simulink model "BuckyWagon_01"  (Simulink 7.5)
settings: Solver=FixedStepDiscrete  StartTime=0.0  StopTime=10.0  RelTol=1e-3
PreLoadFcn:
  | try, eval([bdroot '_setup']); catch, eval('model_setup', ''); end
InitFcn:
  | try, eval([bdroot '_setup']); catch, eval('model_setup', ''); end
undefined symbols (not defined in the file or in its folder): ECU565, High, Low, miniviewSetup, motohawk_build_version, motohawk_get_faults, motohawk_setup_toolchains, motohawk_trunc_name, motohawk_vardec_config_group, motohawk_vardec_path, tc, True
libraries: MotoHawk_lib x406, simulink x30, miniview_lib x10, motohawk_control_primitives_lib x9, MotoHawk_VDOGauge_lib x8, motohawk_engine_lib x7, motohawk_annotations_lib x2
(part 3 of 7)

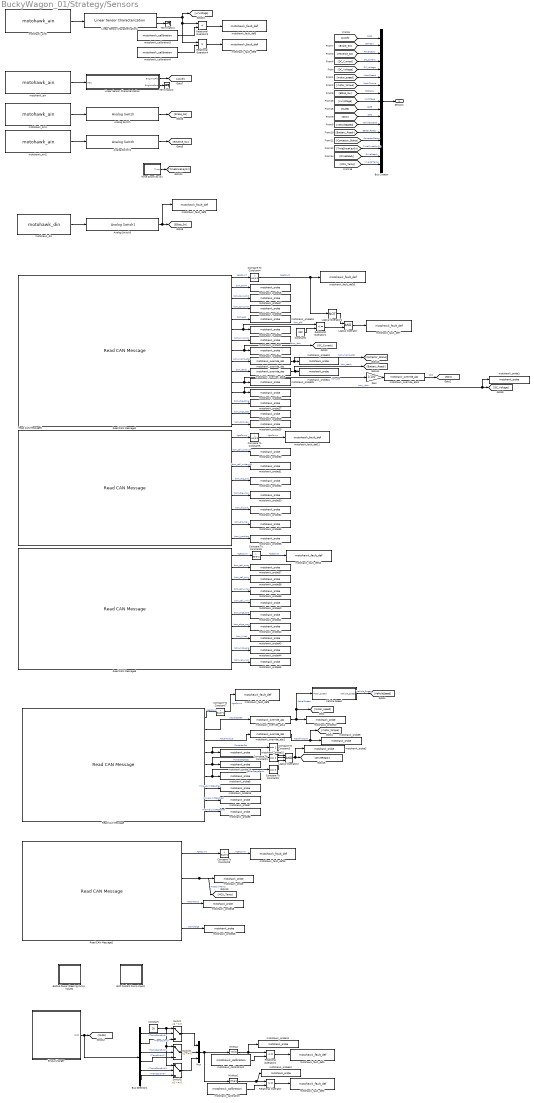
== system BuckyWagon_01/Strategy/Sensors ==
  Analog Switch : motohawk_engine_lib/Analog Switch  SystemSampleTime=-1  nam='Brake_Switch'  prefix='Brake_'  switchpoint=500  polarity=High-True  parent_group='Sensors | Brake'
  Analog Switch1 : motohawk_engine_lib/Analog Switch  SystemSampleTime=-1  nam='Reverse_Switch'  prefix='Reverse_'  switchpoint=500  polarity=Low-True  parent_group='Sensors | Reverse'
  Analog Switch3 : motohawk_engine_lib/Analog Switch1  SystemSampleTime=-1  nam='EStop_Switch'  prefix='EStop_'  polarity=Low-True  parent_group='Sensors | EStop'
  Brusa Charger : Subsystem  AncestorBlock=motohawk_annotations_lib/Display Image File  mask(Display Image File){image_file='NLG5.jpg'}
      mask prompts: image_file "Image File"
      mask help:
      | Enter an image file on the current MATLAB path to display on this block.
      |
      | Double-clicking this block opens the contents of the subsystem.  Right-click and select 'Mask parameters...' to select a new image file.
      |
      | To use just the mask of this block in a model, but supply your own contents, break the link to the library.
      mask init:
      | try,
      | 	img = imread(image_file);
      | 	motohawk_block_image(gcb, image_file);
      | catch,
      | 	img = imread('image_not_found.jpg');
      | end
      settings: OpenFcn=open_system(gcb,'force');  MoveFcn=motohawk_block_image(gcb, motohawk_get_param_ws(gcb, 'image_file'));
      mask Display: image(img);
  Bus Creator : BusCreator  Inputs=17
  Bus Selector1 : BusSelector  OutputSignals=Errors/Warnings.TempSensExt1,Temp.TempExtrn1,Errors/Warnings.TempSensExt2,Temp.TempExtrn2,Errors/Warnings.TempSensExt3,Temp.TempExtrn3
  Compare To Constant1 : simulink/Logic and Bit Operations/Compare To Constant  SystemSampleTime=-1  relop===  const=1  LogicOutDataTypeMode=boolean
  Compare To Constant3 : simulink/Logic and Bit Operations/Compare To Constant  SystemSampleTime=-1  relop===  const=1  LogicOutDataTypeMode=boolean
  Compare To Constant{4..8} (5 alike) : simulink/Logic and Bit Operations/Compare To Constant  SystemSampleTime=-1  relop=>  const=50/5*2  LogicOutDataTypeMode=boolean  ZeroCross=off
  Compare To Constant9 : simulink/Logic and Bit Operations/Compare To Constant  SystemSampleTime=-1  relop===  const=0  LogicOutDataTypeMode=boolean
  Constant : Constant  Value=20  OutDataType=sfix(16)  OutScaling=2^0
  Constant1 : Constant  Value=200  OutDataType=fixdt(1, 16)  OutScaling=2^0
  EHPAS Power Steering Pump Inputts : Subsystem  TreatAsAtomicUnit=on
  EMP Coolant Pump Inputs : Subsystem  TreatAsAtomicUnit=on
  Gain : Gain  Gain=1/100  ParameterDataType=fixdt(1, 16)  ParameterScaling=2^0  OutDataType=fixdt(1, 16)  OutScaling=2^0
  Linear Sensor Characterization : Subsystem  AncestorBlock=motohawk_engine_lib/Linear Sensor Characterization  mask(Linear Sensor Characterization){nam='Accel_Pedal', prefix='Accel_', units='%', inputunits='ADC', parent_group='Sensors | Accel', samp_time=0.005}
      mask prompts: nam "Name"; units "Output Units"; inputunits "Input Units"; parent_group "MotoTune Group"; samp_time "Sample Time"
      mask help:
      | Converts from A/D Counts to Engineering Units, using a Gain and Offset.
      | Saturates the converted value around Min and Max values, and triggers a Fault when out of range.
      mask init:
      | lbl = ['Linear Sensor: ' nam ' [' units ']'];
      | group = [parent_group ' | ' nam];
      settings: RTWSystemCode=Function  RTWFcnNameOpts=Use subsystem name  RTWFileNameOpts=Use function name
      mask Display:
      | patch([0 0 1 1], [0 0.075 0.075 0], [230/255 0/255 0/255])
      | patch([0 0 1 1], [0.025 0.05 0.05 0.025], [150/255 0/255 0/255])
      | patch([0 0 1 1], [0 0.025 0.025 0], [0/255 0/255 0/255])
      | 
      | disp(lbl);
  Linear Sensor Characterization1 : motohawk_engine_lib/Linear Sensor Characterization  SystemSampleTime=-1  nam='LVVolt'  prefix='LVVolt_'  units='V'  inputunits='ADC'  parent_group='Sensors | LVVolt'  samp_time=0.005
      link override First Order Low Pass/motohawk_calibration: val=0.01
      link override motohawk_calibration3: val=0.69
      link override motohawk_calibration4: val=0.041379
      link override motohawk_fault_def2: id=0
      link override motohawk_fault_def3: id=0
  Logical Operator : Logic  AllPortsSameDT=off  OutDataTypeMode=boolean  LogicDataType=fixdt(0, 8)  OutDataTypeStr=boolean
  Logical Operator1 : Logic  Operator=NOT  Inputs=1  AllPortsSameDT=off  OutDataTypeMode=boolean  LogicDataType=fixdt(0, 8)  OutDataTypeStr=boolean
  Logical Operator2 : Logic  Inputs=3  IconShape=distinctive  AllPortsSameDT=off  OutDataTypeMode=boolean  LogicDataType=fixdt(0, 8)  OutDataTypeStr=boolean
  MinMax : MinMax  OutDataType=sfix(16)  OutScaling=2^0
  MinMax1 : MinMax  Function=max  OutDataType=sfix(16)  OutScaling=2^0
  Mux : Mux  Inputs=3
  Read CAN Message : MotoHawk_lib/CAN Blocks/Read CAN Message  nam=['CAN_' num2str(2)]  bus=-2  msg=solectria_CANStatusID1  queue=1  slot=''  valid=off  stale=on  labelwires=on
  Read CAN Message1 : MotoHawk_lib/CAN Blocks/Read CAN Message  nam='CAN_2'  bus=-2  msg=BMS_A123_410  queue=1  slot=''  valid=off  stale=on  labelwires=on
  Read CAN Message2 : MotoHawk_lib/CAN Blocks/Read CAN Message  nam=['CAN_' num2str(2)]  bus=-2  msg=solectria_CANStatusID2  queue=1  slot=''  valid=off  stale=on  labelwires=on
  Read CAN Message5 : MotoHawk_lib/CAN Blocks/Read CAN Message  nam='CAN_2'  bus=-2  msg=BMS_A123_420  queue=1  slot=''  valid=off  stale=on  labelwires=on
  Read CAN Message6 : MotoHawk_lib/CAN Blocks/Read CAN Message  nam='CAN_2'  bus=-2  msg=BMS_A123_430  queue=1  slot=''  valid=off  stale=on  labelwires=on
  Relational Operator : RelationalOperator  LogicOutDataTypeMode=boolean  OutDataTypeStr=boolean
  Relational Operator1 : RelationalOperator  Operator=<=  LogicOutDataTypeMode=boolean  LogicDataType=fixdt(0, 8)  OutDataTypeStr=boolean
  Relational Operator2 : RelationalOperator  Operator=<=  LogicOutDataTypeMode=boolean  OutDataTypeStr=boolean
  Relational Operator3 : RelationalOperator  Operator=<  LogicOutDataTypeMode=boolean  OutDataTypeStr=boolean
  Relational Operator4 : RelationalOperator  Operator=>  LogicOutDataTypeMode=boolean  OutDataTypeStr=boolean
  Switch : Switch  Criteria=u2 ~= 0  OutDataType=sfix(16)  OutScaling=2^0
  Switch1 : Switch  Criteria=u2 ~= 0  OutDataType=sfix(16)  OutScaling=2^0
  Switch2 : Switch  Criteria=u2 ~= 0  OutDataType=sfix(16)  OutScaling=2^0
  Terminator2 : Terminator
  Terminator4 : Terminator
  Time Since Key On : Subsystem
  Vehicle Speed : Subsystem
  motohawk_ain : MotoHawk_lib/Analog I//O Blocks/motohawk_ain  res_name=[]  text_resource=AN4M  code_resource=NONE  val_resource=-1  target=ECU565-128  resource_enum_str=(None)=-1,ECUP=53,DRVP=54,XDRP=55,AN1M=56,AN2M=57,AN3M=58,AN4M=59,AN5M=60,AN6M=61,AN7M=62,AN8M=63,AN9M=64,AN10M=65,AN11M=66,AN12M=67,AN13M=68,AN14M=69,AN15M=70,AN16M=71,AN17M=72,AN18M=73,AN19M=74,AN20M=75,AN21M=76,AN22M=77,AN23M=78,AN24M=79,AN25M=80,AN26M=81,AN27M=82,AN28M=83,AN29M=84,AN30M=85,AN31M=86,AN32M=87,AN33M=88,AN34M=89,O2A=90,O2B=91,XDRP_B=92,REF_14V=143  altref=5V Reference  typ=uint16  num_adc_bits=10  use_stat=off  use_vardec=on  nam='Accel_Pedal_Pin'  read_level=1  write_level=1  group='System | I/O Pins | Inputs Config'
  motohawk_ain1 : MotoHawk_lib/Analog I//O Blocks/motohawk_ain  res_name=[]  text_resource=AN2M  code_resource=NONE  val_resource=-1  target=ECU565-128  resource_enum_str=(None)=-1,ECUP=53,DRVP=54,XDRP=55,AN1M=56,AN2M=57,AN3M=58,AN4M=59,AN5M=60,AN6M=61,AN7M=62,AN8M=63,AN9M=64,AN10M=65,AN11M=66,AN12M=67,AN13M=68,AN14M=69,AN15M=70,AN16M=71,AN17M=72,AN18M=73,AN19M=74,AN20M=75,AN21M=76,AN22M=77,AN23M=78,AN24M=79,AN25M=80,AN26M=81,AN27M=82,AN28M=83,AN29M=84,AN30M=85,AN31M=86,AN32M=87,AN33M=88,AN34M=89,O2A=90,O2B=91,XDRP_B=92,REF_14V=143  altref=5V Reference  typ=uint16  num_adc_bits=10  use_stat=off  use_vardec=on  nam='Brake_Switch_Pin'  read_level=1  write_level=1  group='System | I/O Pins | Inputs Config'
  motohawk_ain2 : MotoHawk_lib/Analog I//O Blocks/motohawk_ain  res_name=[]  text_resource=AN1M  code_resource=NONE  val_resource=-1  target=ECU565-128  resource_enum_str=(None)=-1,ECUP=53,DRVP=54,XDRP=55,AN1M=56,AN2M=57,AN3M=58,AN4M=59,AN5M=60,AN6M=61,AN7M=62,AN8M=63,AN9M=64,AN10M=65,AN11M=66,AN12M=67,AN13M=68,AN14M=69,AN15M=70,AN16M=71,AN17M=72,AN18M=73,AN19M=74,AN20M=75,AN21M=76,AN22M=77,AN23M=78,AN24M=79,AN25M=80,AN26M=81,AN27M=82,AN28M=83,AN29M=84,AN30M=85,AN31M=86,AN32M=87,AN33M=88,AN34M=89,O2A=90,O2B=91,XDRP_B=92,REF_14V=143  altref=5V Reference  typ=uint16  num_adc_bits=10  use_stat=off  use_vardec=on  nam='Reverse_Switch_Pin'  read_level=1  write_level=1  group='System | I/O Pins | Inputs Config'
  motohawk_ain5 : MotoHawk_lib/Analog I//O Blocks/motohawk_ain  res_name=[]  text_resource=DRVP  code_resource=NONE  val_resource=-1  target=ECU565-128  resource_enum_str=(None)=-1,ECUP=53,DRVP=54,XDRP=55,AN1M=56,AN2M=57,AN3M=58,AN4M=59,AN5M=60,AN6M=61,AN7M=62,AN8M=63,AN9M=64,AN10M=65,AN11M=66,AN12M=67,AN13M=68,AN14M=69,AN15M=70,AN16M=71,AN17M=72,AN18M=73,AN19M=74,AN20M=75,AN21M=76,AN22M=77,AN23M=78,AN24M=79,AN25M=80,AN26M=81,AN27M=82,AN28M=83,AN29M=84,AN30M=85,AN31M=86,AN32M=87,AN33M=88,AN34M=89,O2A=90,O2B=91,XDRP_B=92,REF_14V=143  altref=5V Reference  typ=uint16  num_adc_bits=10  use_stat=off  use_vardec=on  nam='LV_Voltage_Pin'  read_level=1  write_level=1  group='System | I/O Pins | Inputs Config'
  motohawk_calibration : MotoHawk_lib/Calibration & Probing Blocks/motohawk_calibration  nam='BattOverTemp_Pt'  val=70  storage=Calibration  show_more=on  name_source=Use Parameter  data_type=Inherit from 'Default Value'  read_level=1  write_level=1  ovr_cals=on  view_as=Number  enum_struct={'Disabled', 'Enabled'}  vector_style=Wide Row  use_help_units=on  help='Temperature at which an overtemp fault occurs'  units='C'  use_header_enum=off  row_header_enum={}  col_header_enum={}  use_min_max=off  min_val=-inf  max_val=inf  use_precision=off  precision=''  gain=1  offset=0  exp=1  use_mototune_group=on  mototune_group='Sensors | Brusa'
  motohawk_calibration2 : MotoHawk_lib/Calibration & Probing Blocks/motohawk_calibration  nam='BattUnderTemp_Pt'  val=-40  storage=Calibration  show_more=on  name_source=Use Parameter  data_type=Inherit from 'Default Value'  read_level=1  write_level=1  ovr_cals=on  view_as=Number  enum_struct={'Disabled', 'Enabled'}  vector_style=Wide Row  use_help_units=on  help='Temperature at which an overtemp fault occurs'  units='C'  use_header_enum=off  row_header_enum={}  col_header_enum={}  use_min_max=off  min_val=-inf  max_val=inf  use_precision=off  precision=''  gain=1  offset=0  exp=1  use_mototune_group=on  mototune_group='Sensors | Brusa'
  motohawk_calibration3 : MotoHawk_lib/Calibration & Probing Blocks/motohawk_calibration  nam='Low12VThres'  val=12.8  storage=Calibration  show_more=on  name_source=Use Parameter  data_type=Inherit from 'Default Value'  read_level=1  write_level=1  ovr_cals=on  view_as=Number  enum_struct={'Disabled', 'Enabled'}  vector_style=Wide Row  use_help_units=on  help='Voltage below with low 12V fault occurs.'  units='V'  use_header_enum=off  row_header_enum={}  col_header_enum={}  use_min_max=off  min_val=-inf  max_val=inf  use_precision=on  precision=''  gain=1  offset=0  exp=1  use_mototune_group=on  mototune_group='Sensors | LVVolt'
  motohawk_calibration4 : MotoHawk_lib/Calibration & Probing Blocks/motohawk_calibration  nam='High12VThres'  val=14.5  storage=Calibration  show_more=on  name_source=Use Parameter  data_type=Inherit from 'Default Value'  read_level=1  write_level=1  ovr_cals=on  view_as=Number  enum_struct={'Disabled', 'Enabled'}  vector_style=Wide Row  use_help_units=on  help='Voltage below with low 12V fault occurs.'  units='V'  use_header_enum=off  row_header_enum={}  col_header_enum={}  use_min_max=off  min_val=-inf  max_val=inf  use_precision=on  precision=''  gain=1  offset=0  exp=1  use_mototune_group=on  mototune_group='Sensors | LVVolt'
  motohawk_din : MotoHawk_lib/Digital I//O Blocks/motohawk_din  resource_name=[]  text_resource=(None)  code_resource=RES_AN1M  val_resource=-1  target=ECU565-128  resource_enum_str=(None)=-1,AN1M=56,AN2M=57,AN3M=58,AN4M=59,AN5M=60,AN6M=61,AN7M=62,AN8M=63,AN9M=64,AN10M=65,AN11M=66,AN12M=67,AN13M=68,AN14M=69,AN15M=70,AN16M=71,AN17M=72,AN18M=73,AN19M=74,AN20M=75,AN21M=76,AN22M=77,AN23M=78,AN24M=79,AN25M=80,AN26M=81,AN27M=82,AN28M=83,AN29M=84,AN30M=85,AN31M=86,AN32M=87,AN33M=88,AN34M=89,O2A=90,O2B=91,DG1M=93,DG2M=94,DG3M=95,DG4M=96,DG5M=102,DG6M=103,DG7M=104,SPD1=105,SPD2=106,DG8M=111  pullup=None  use_stat=off  use_vardec=on  nam='EStop_Switch_Pin'  read_level=1  write_level=1  group='System | I/O Pins | Inputs Config'
  motohawk_fault_def10 : MotoHawk_lib/Fault Management Blocks/motohawk_fault_def  nam='NoCAN_BCM_410'  mode=Enabled  id=0  x=10  y=20  input_suspected=on  indeterminate=off  increment_xy=on  downsample_count=1  ovr_cals=on  ovr_actions=on  show_actions=off  action1_name=''  action1_cond=(None)  action2_name=''  action2_cond=(None)  action3_name=''  action3_cond=(None)  action4_name=''  action4_cond=(None)
  motohawk_fault_def11 : MotoHawk_lib/Fault Management Blocks/motohawk_fault_def  nam='NoCAN_BCM_420'  mode=Enabled  id=0  x=10  y=20  input_suspected=on  indeterminate=off  increment_xy=on  downsample_count=1  ovr_cals=on  ovr_actions=on  show_actions=off  action1_name=''  action1_cond=(None)  action2_name=''  action2_cond=(None)  action3_name=''  action3_cond=(None)  action4_name=''  action4_cond=(None)
  motohawk_fault_def12 : MotoHawk_lib/Fault Management Blocks/motohawk_fault_def  nam='NoCAN_BCM_430'  mode=Enabled  id=0  x=10  y=20  input_suspected=on  indeterminate=off  increment_xy=on  downsample_count=1  ovr_cals=on  ovr_actions=on  show_actions=off  action1_name=''  action1_cond=(None)  action2_name=''  action2_cond=(None)  action3_name=''  action3_cond=(None)  action4_name=''  action4_cond=(None)
  motohawk_fault_def13 : MotoHawk_lib/Fault Management Blocks/motohawk_fault_def  nam='NoCAN_Solectria_462'  mode=Enabled  id=[]  x=50/5  y=50/5*2  input_suspected=on  indeterminate=off  increment_xy=on  downsample_count=1  ovr_cals=on  ovr_actions=on  show_actions=off  action1_name=''  action1_cond=(None)  action2_name=''  action2_cond=(None)  action3_name=''  action3_cond=(None)  action4_name=''  action4_cond=(None)
  motohawk_fault_def2 : MotoHawk_lib/Fault Management Blocks/motohawk_fault_def  nam='BattOverTemp'  mode=Disabled  id=0  x=25  y=50  input_suspected=on  indeterminate=off  increment_xy=on  downsample_count=1  ovr_cals=on  ovr_actions=on  show_actions=off  action1_name=''  action1_cond=(None)  action2_name=''  action2_cond=(None)  action3_name=''  action3_cond=(None)  action4_name=''  action4_cond=(None)
  motohawk_fault_def3 : MotoHawk_lib/Fault Management Blocks/motohawk_fault_def  nam='ESTOPped'  mode=Sticky  id=0  x=50  y=100  input_suspected=on  indeterminate=off  increment_xy=on  downsample_count=1  ovr_cals=on  ovr_actions=on  show_actions=off  action1_name='DisableDrive'  action1_cond=Active  action2_name=''  action2_cond=(None)  action3_name=''  action3_cond=(None)  action4_name=''  action4_cond=(None)
  motohawk_fault_def4 : MotoHawk_lib/Fault Management Blocks/motohawk_fault_def  nam='BattUnderTemp'  mode=Disabled  id=0  x=25  y=50  input_suspected=on  indeterminate=off  increment_xy=on  downsample_count=1  ovr_cals=on  ovr_actions=on  show_actions=off  action1_name=''  action1_cond=(None)  action2_name=''  action2_cond=(None)  action3_name=''  action3_cond=(None)  action4_name=''  action4_cond=(None)
  motohawk_fault_def5 : MotoHawk_lib/Fault Management Blocks/motohawk_fault_def  nam='LVVoltLow'  mode=Enabled  id=0  x=100  y=200  input_suspected=on  indeterminate=off  increment_xy=on  downsample_count=1  ovr_cals=on  ovr_actions=on  show_actions=off  action1_name=''  action1_cond=(None)  action2_name=''  action2_cond=(None)  action3_name=''  action3_cond=(None)  action4_name=''  action4_cond=(None)
  motohawk_fault_def6 : MotoHawk_lib/Fault Management Blocks/motohawk_fault_def  nam='LVVoltHigh'  mode=Enabled  id=0  x=25  y=50  input_suspected=on  indeterminate=off  increment_xy=on  downsample_count=1  ovr_cals=on  ovr_actions=on  show_actions=off  action1_name=''  action1_cond=(None)  action2_name=''  action2_cond=(None)  action3_name=''  action3_cond=(None)  action4_name=''  action4_cond=(None)
  motohawk_fault_def7 : MotoHawk_lib/Fault Management Blocks/motohawk_fault_def  nam='GroundFlt'  mode=Sticky  id=0  x=25  y=50  input_suspected=on  indeterminate=off  increment_xy=on  downsample_count=1  ovr_cals=on  ovr_actions=on  show_actions=off  action1_name='EmergencyShutdown'  action1_cond=Active  action2_name=''  action2_cond=(None)  action3_name=''  action3_cond=(None)  action4_name=''  action4_cond=(None)
  motohawk_fault_def8 : MotoHawk_lib/Fault Management Blocks/motohawk_fault_def  nam='NoCAN_Solectria_461'  mode=Enabled  id=[]  x=50/5  y=50/5*2  input_suspected=on  indeterminate=off  increment_xy=on  downsample_count=1  ovr_cals=on  ovr_actions=on  show_actions=off  action1_name=''  action1_cond=(None)  action2_name=''  action2_cond=(None)  action3_name=''  action3_cond=(None)  action4_name=''  action4_cond=(None)
  motohawk_override_abs : MotoHawk_lib/Calibration & Probing Blocks/motohawk_override_abs  SystemSampleTime=-1  parent_name='bcm_mainc_stat'  parent_val=0  show_more=on  name_source=Use Parameter  parent_read_level=1  parent_override_level=1  view_as=Number  enum_struct={'Disabled', 'Enabled'}  use_help_units=off  parent_help=''  parent_units=''  use_min_max=off  parent_min=-inf  parent_max=inf  use_precision=off  parent_precision=''  parent_gain=1  parent_offset=0  parent_exp=1  use_mototune_group=on  parent_group='Sensors | BCM'
  motohawk_override_abs1 : MotoHawk_lib/Calibration & Probing Blocks/motohawk_override_abs  SystemSampleTime=-1  parent_name='Override_Absolute'  parent_val=0  show_more=on  name_source=Use Input Wire Name  parent_read_level=1  parent_override_level=1  view_as=Number  enum_struct={'Disabled', 'Enabled'}  use_help_units=off  parent_help=''  parent_units=''  use_min_max=off  parent_min=-inf  parent_max=inf  use_precision=off  parent_precision=''  parent_gain=1  parent_offset=0  parent_exp=1  use_mototune_group=on  parent_group='Sensors | Solectria'
  motohawk_override_abs2 : MotoHawk_lib/Calibration & Probing Blocks/motohawk_override_abs  SystemSampleTime=-1  parent_name='Override_Absolute'  parent_val=0  show_more=on  name_source=Use Input Wire Name  parent_read_level=1  parent_override_level=1  view_as=Number  enum_struct={'Disabled', 'Enabled'}  use_help_units=off  parent_help=''  parent_units=''  use_min_max=off  parent_min=-inf  parent_max=inf  use_precision=off  parent_precision=''  parent_gain=1  parent_offset=0  parent_exp=1  use_mototune_group=on  parent_group='Sensors | Solectria'
  motohawk_override_abs4 : MotoHawk_lib/Calibration & Probing Blocks/motohawk_override_abs  SystemSampleTime=-1  parent_name='SOC'  parent_val=0.5  show_more=on  name_source=Use Parameter  parent_read_level=1  parent_override_level=1  view_as=Number  enum_struct={'Disabled', 'Enabled'}  use_help_units=off  parent_help=''  parent_units=''  use_min_max=on  parent_min=0  parent_max=1  use_precision=off  parent_precision=''  parent_gain=1  parent_offset=0  parent_exp=1  use_mototune_group=on  parent_group='Sensors | BCM'
  motohawk_override_abs5 : MotoHawk_lib/Calibration & Probing Blocks/motohawk_override_abs  SystemSampleTime=-1  parent_name='bcm_ready'  parent_val=0  show_more=on  name_source=Use Parameter  parent_read_level=1  parent_override_level=1  view_as=Number  enum_struct={'Disabled', 'Enabled'}  use_help_units=off  parent_help=''  parent_units=''  use_min_max=off  parent_min=-inf  parent_max=inf  use_precision=off  parent_precision=''  parent_gain=1  parent_offset=0  parent_exp=1  use_mototune_group=on  parent_group='Sensors | BCM'
  motohawk_probe{,6..8,13..15,48} (8 alike) : MotoHawk_lib/Calibration & Probing Blocks/motohawk_probe  nam='Probe'  show_more=on  name_source=Use Input Wire Name  read_level=1  view_as=Number  enum_struct={'Disabled', 'Enabled'}  vector_style=Wide Row  use_help_units=off  help=''  units=''  use_header_enum=off  row_header_enum={}  col_header_enum={}  use_precision=off  precision=''  gain=1  offset=0  exp=1  use_mototune_group=on  mototune_group='Sensors | Solectria'
  motohawk_probe1 : MotoHawk_lib/Calibration & Probing Blocks/motohawk_probe  nam='DC_Voltage'  show_more=on  name_source=Use Parameter  read_level=1  view_as=Number  enum_struct={'Disabled', 'Enabled'}  vector_style=Wide Row  use_help_units=off  help=''  units=''  use_header_enum=off  row_header_enum={}  col_header_enum={}  use_precision=off  precision=''  gain=1  offset=0  exp=1  use_mototune_group=on  mototune_group='Sensors'
  motohawk_probe10 : MotoHawk_lib/Calibration & Probing Blocks/motohawk_probe  nam='Probe'  show_more=on  name_source=Use Input Wire Name  read_level=1  view_as=Number  enum_struct={'Disabled', 'Enabled'}  vector_style=Wide Row  use_help_units=off  help=''  units=''  use_header_enum=off  row_header_enum={}  col_header_enum={}  use_precision=off  precision=''  gain=1  offset=0  exp=1  use_mototune_group=on  mototune_group='Sensors'
  motohawk_probe11 : MotoHawk_lib/Calibration & Probing Blocks/motohawk_probe  nam='BattMinTemp'  show_more=on  name_source=Use Parameter  read_level=1  view_as=Number  enum_struct={'Disabled', 'Enabled'}  vector_style=Wide Row  use_help_units=off  help=''  units=''  use_header_enum=off  row_header_enum={}  col_header_enum={}  use_precision=off  precision=''  gain=1  offset=0  exp=1  use_mototune_group=on  mototune_group='Sensors | Brusa'
  motohawk_probe12 : MotoHawk_lib/Calibration & Probing Blocks/motohawk_probe  nam='BattMaxTemp'  show_more=on  name_source=Use Parameter  read_level=1  view_as=Number  enum_struct={'Disabled', 'Enabled'}  vector_style=Wide Row  use_help_units=off  help=''  units=''  use_header_enum=off  row_header_enum={}  col_header_enum={}  use_precision=off  precision=''  gain=1  offset=0  exp=1  use_mototune_group=on  mototune_group='Sensors | Brusa'
  motohawk_probe{16..45} (30 alike) : MotoHawk_lib/Calibration & Probing Blocks/motohawk_probe  nam='Probe'  show_more=on  name_source=Use Input Wire Name  read_level=1  view_as=Number  enum_struct={'Disabled', 'Enabled'}  vector_style=Wide Row  use_help_units=off  help=''  units=''  use_header_enum=off  row_header_enum={}  col_header_enum={}  use_precision=off  precision=''  gain=1  offset=0  exp=1  use_mototune_group=on  mototune_group='Sensors | BCM'
  motohawk_probe2 : MotoHawk_lib/Calibration & Probing Blocks/motohawk_probe  nam='DriveReady'  show_more=on  name_source=Use Parameter  read_level=1  view_as=Number  enum_struct={'Disabled', 'Enabled'}  vector_style=Wide Row  use_help_units=off  help=''  units=''  use_header_enum=off  row_header_enum={}  col_header_enum={}  use_precision=off  precision=''  gain=1  offset=0  exp=1  use_mototune_group=on  mototune_group='Sensors'
  motohawk_probe46 : MotoHawk_lib/Calibration & Probing Blocks/motohawk_probe  nam='DCVoltage_Solectria'  show_more=on  name_source=Use Parameter  read_level=1  view_as=Number  enum_struct={'Disabled', 'Enabled'}  vector_style=Wide Row  use_help_units=off  help=''  units=''  use_header_enum=off  row_header_enum={}  col_header_enum={}  use_precision=off  precision=''  gain=1  offset=0  exp=1  use_mototune_group=on  mototune_group='Sensors | Solectria'
  motohawk_probe9 : MotoHawk_lib/Calibration & Probing Blocks/motohawk_probe  nam='Probe'  show_more=on  name_source=Use Input Wire Name  read_level=1  view_as=Number  enum_struct={'Disabled', 'Enabled'}  vector_style=Wide Row  use_help_units=off  help=''  units=''  use_header_enum=off  row_header_enum={}  col_header_enum={}  use_precision=off  precision=''  gain=1  offset=0  exp=1  use_mototune_group=on  mototune_group='Sensors'
  Sensors : Outport  OutDataType=sfix(16)  OutScaling=2^0
  wires:
  motohawk_ain/1 -> Linear Sensor Characterization/1(ADC)
  motohawk_ain1/1 -> Analog Switch/1
  Analog Switch/1 -> [Brake_Sw]
  Linear Sensor Characterization/1(EngUnitsFilt) -> [Accel]
  Linear Sensor Characterization/2(EngUnitsRaw) -> Terminator2/1
  Bus Creator/1 -> Sensors/1
  [Accel] -> Bus Creator/1  "Accel"
  [Brake_Sw] -> Bus Creator/2  "BrakeSw"
  [Reverse_Sw] -> Bus Creator/3  "ReverseSw"
  motohawk_ain2/1 -> Analog Switch1/1
  Analog Switch1/1 -> [Reverse_Sw]
  motohawk_din/1 -> Analog Switch3/1
  Analog Switch3/1 -> [EStop_Sw], motohawk_fault_def3/1
  motohawk_ain5/1 -> Linear Sensor Characterization1/1
  Linear Sensor Characterization1/2 -> Terminator4/1
  motohawk_calibration3/1 -> Relational Operator3/2
  Linear Sensor Characterization1/1 -> [LVVoltage], Relational Operator3/1, Relational Operator4/1
  Relational Operator3/1 -> motohawk_fault_def5/1
  motohawk_calibration4/1 -> Relational Operator4/2
  Relational Operator4/1 -> motohawk_fault_def6/1
  [DC_Current] -> Bus Creator/4  "DC_Current"
  [DC_Voltage] -> Bus Creator/5  "DC_Voltage"
  [motor_speed] -> Bus Creator/6  "MotorSpeed"
  [motor_torque] -> Bus Creator/7  "MotorTorque"
  [EStop_Sw] -> Bus Creator/8  "EStopSw"
  [LVVoltage] -> Bus Creator/9  "LVVoltage"
  [NLG5] -> Bus Creator/10  "NLG5"
  [SOC] -> Bus Creator/11  "SOC"
  [VehicleSpeed] -> Bus Creator/12  "VehicleSpeed"
  [Contactor_Status] -> Bus Creator/14  "ContactorStatus"
  [Battery_Ready] -> Bus Creator/13  "BatteryReady"
  Time Since Key On/1(Time) -> [TimeSinceKeyOn]
  [TimeSinceKeyOn] -> Bus Creator/15  "TimeSinceKeyOn"
  [DriveReady] -> Bus Creator/16  "DriveReady"
  [MCU_Temp] -> Bus Creator/17  "InverterTemp"
  Read CAN Message1/2 -> motohawk_probe16/1  "bcm_alarm"
  Read CAN Message1/3 -> motohawk_probe17/1  "bcm_cpwr_cmd"
  Read CAN Message1/4 -> motohawk_probe18/1  "bcm_cpwr_mon"
  Read CAN Message1/5 -> motohawk_probe19/1  "bcm_epo"
  Read CAN Message1/6 -> motohawk_probe20/1, Relational Operator1/1  "bcm_gfd"
  Read CAN Message1/7 -> motohawk_probe21/1  "bcm_hvil_mon"
  Read CAN Message1/8 -> motohawk_probe22/1, [DC_Current]  "bcm_ibat"
  Read CAN Message1/9 -> motohawk_override_abs/1  "bcm_mainc_stat"
  Read CAN Message1/10 -> motohawk_override_abs5/1  "bcm_ready"
  Read CAN Message1/11 -> motohawk_probe25/1, Gain/1  "bcm_soc"
  Read CAN Message1/12 -> motohawk_probe26/1, [DC_Voltage], motohawk_probe1/1  "bcm_vbat"
  Read CAN Message1/13 -> motohawk_probe27/1  "bcm_chg_done"
  Read CAN Message1/14 -> motohawk_probe28/1  "bcm_chgc_stat"
  Read CAN Message1/15 -> motohawk_probe29/1  "bcm_cool_req"
  Read CAN Message5/2 -> motohawk_probe30/1  "bcm_cell_overvolt"
  Read CAN Message5/3 -> motohawk_probe31/1  "bcm_cell_undervolt"
  Read CAN Message5/4 -> motohawk_probe32/1  "bcm_chg_buf"
  Read CAN Message5/5 -> motohawk_probe33/1  "bcm_chg_max"
  Read CAN Message5/6 -> motohawk_probe34/1  "bcm_dis_buf"
  Read CAN Message5/7 -> motohawk_probe35/1  "bcm_dis_max"
  Read CAN Message5/8 -> motohawk_probe36/1  "bcm_t_coolant"
  Read CAN Message6/2 -> motohawk_probe37/1  "bcm_cell_tmax"
  Read CAN Message6/3 -> motohawk_probe38/1  "bcm_cell_tmin"
  Read CAN Message6/4 -> motohawk_probe39/1  "bcm_cell_vmax"
  Read CAN Message6/5 -> motohawk_probe40/1  "bcm_cell_vmin"
  Read CAN Message6/6 -> motohawk_probe41/1  "bcm_chga_ena"
  Read CAN Message6/7 -> motohawk_probe42/1  "bcm_chga_mon"
  Read CAN Message6/8 -> motohawk_probe43/1  "bcm_lvbat"
  Read CAN Message6/9 -> motohawk_probe44/1  "bcm_mod_ena"
  Read CAN Message6/10 -> motohawk_probe45/1  "bcm_veh_mon"
  Compare To Constant4/1 -> motohawk_fault_def10/1, Logical Operator1/1  "AgeCount"
  Read CAN Message1/1 -> Compare To Constant4/1  "AgeCount"
  Compare To Constant5/1 -> motohawk_fault_def11/1  "AgeCount"
  Read CAN Message5/1 -> Compare To Constant5/1  "AgeCount"
  Compare To Constant6/1 -> motohawk_fault_def12/1  "AgeCount"
  Read CAN Message6/1 -> Compare To Constant6/1  "AgeCount"
  Constant1/1 -> Relational Operator1/2
  motohawk_override_abs4/1 -> [SOC]  "SOC"
  Gain/1 -> motohawk_override_abs4/1
  Relational Operator1/1 -> Logical Operator/2
  Logical Operator/1 -> motohawk_fault_def7/1
  Logical Operator1/1 -> Logical Operator/1
  motohawk_override_abs/1 -> motohawk_probe23/1, [Contactor_Status]  "bcm_mainc_stat"
  motohawk_override_abs5/1 -> [Battery_Ready], motohawk_probe24/1  "bcm_ready"
  Read CAN Message/3 -> motohawk_override_abs2/1  "ActualTorque"
  Read CAN Message/4 -> motohawk_probe15/1, Compare To Constant3/1  "ContactorSts"
  Read CAN Message/5 -> motohawk_probe14/1, Compare To Constant1/1  "PowerStageSts"
  Read CAN Message/6 -> motohawk_probe8/1, Compare To Constant9/1  "PowerStageFault"
  Read CAN Message/7 -> motohawk_probe13/1  "TorqueLimitReached"
  Read CAN Message/8 -> motohawk_probe7/1  "PowerLimitReached"
  Read CAN Message/9 -> motohawk_probe6/1  "ThermalLimitReached"
  Read CAN Message/1 -> Compare To Constant7/1  "AgeCount"
  Compare To Constant7/1 -> motohawk_fault_def8/1  "AgeCount"
  Read CAN Message2/2 -> motohawk_probe/1, [MCU_Temp]  "HeatsinkTemp"
  Read CAN Message2/3 -> motohawk_probe48/1  "MotorTemp"
  Read CAN Message2/1 -> Compare To Constant8/1  "AgeCount"
  motohawk_override_abs1/1 -> motohawk_probe10/1, [motor_speed], Vehicle Speed/1(Motor_Speed)  "ActualSpeed"
  Vehicle Speed/1(Vehicle_Speed) -> [VehicleSpeed]  "Vehicle_Speed"
  Read CAN Message/2 -> motohawk_override_abs1/1  "ActualSpeed"
  motohawk_override_abs2/1 -> motohawk_probe9/1, [motor_torque]  "ActualTorque"
  Read CAN Message2/4 -> motohawk_probe46/1  "DCVoltage"
  Compare To Constant8/1 -> motohawk_fault_def13/1  "AgeCount"
  Compare To Constant1/1 -> Logical Operator2/2
  Compare To Constant3/1 -> Logical Operator2/1
  Compare To Constant9/1 -> Logical Operator2/3
  Logical Operator2/1 -> [DriveReady], motohawk_probe2/1
  Brusa Charger/1(Out1) -> [NLG5], Bus Selector1/1
  MinMax1/1 -> Relational Operator/1, motohawk_probe12/1
  motohawk_calibration/1 -> Relational Operator/2
  Relational Operator/1 -> motohawk_fault_def2/1
  MinMax/1 -> Relational Operator2/1, motohawk_probe11/1
  motohawk_calibration2/1 -> Relational Operator2/2
  Relational Operator2/1 -> motohawk_fault_def4/1
  Bus Selector1/1 -> Switch/2  "<TempSensExt1>"
  Bus Selector1/2 -> Switch/3  "<TempExtrn1>"
  Bus Selector1/3 -> Switch1/2  "<TempSensExt2>"
  Bus Selector1/4 -> Switch1/3  "<TempExtrn2>"
  Bus Selector1/5 -> Switch2/2  "<TempSensExt3>"
  Bus Selector1/6 -> Switch2/3  "<TempExtrn3>"
  Constant/1 -> Switch/1, Switch1/1, Switch2/1
  Switch/1 -> Mux/1
  Switch1/1 -> Mux/2
  Switch2/1 -> Mux/3
  Mux/1 -> MinMax/1, MinMax1/1

== system BuckyWagon_01/Main Power Relay/Background/Delay ==
  note: Delay the rising and falling of a boolean signal
  In : Inport  OutDataType=sfix(16)  OutScaling=2^0
  Constant1 : Constant  Value=0  OutDataType=sfix(16)  OutScaling=2^0  OutDataTypeStr=Inherit: Inherit via back propagation
  Constant2 : Constant  Value=uint16( on_delay_count )  OutDataType=sfix(16)  OutScaling=2^0
  Constant3 : Constant  Value=0  OutDataType=sfix(16)  OutScaling=2^0  OutDataTypeStr=Inherit: Inherit via back propagation
  Constant4 : Constant  Value=uint16( off_delay_count )  OutDataType=sfix(16)  OutScaling=2^0
  Data Type Conversion : DataTypeConversion  RndMeth=Zero
  Data Type Conversion1 : DataTypeConversion  RndMeth=Zero
  Logical Operator : Logic  Operator=NOT  OutDataTypeMode=boolean  OutDataTypeStr=boolean
  Logical Operator1 : Logic  OutDataTypeMode=boolean  OutDataTypeStr=boolean
  Logical Operator2 : Logic  OutDataTypeMode=boolean  OutDataTypeStr=boolean
  MotoHawk S-R Flip-Flop : Subsystem  mask(MotoHawk S-R Flip-Flop){ic_bool=false}
      mask prompts: ic_bool "Initial condition Q (boolean)"
      mask help:
      | When input S (set) is TRUE, output Q is TRUE (and latched until reset).
      | When input R (reset) is TRUE, output Q is FALSE (and latched until set).
      | If both inputs S and R are TRUE, output Q is FALSE (reset wins).
      mask Display:
      | patch([0 0 1 1], [0 0.075 0.075 0], [230/255 0/255 0/255]);
      | patch([0 0 1 1], [0.025 0.05 0.05 0.025], [150/255 0/255 0/255]);
      | patch([0 0 1 1], [0 0.025 0.025 0], [0/255 0/255 0/255])
  Relational Operator1 : RelationalOperator  LogicOutDataTypeMode=boolean  OutDataTypeStr=boolean  ZeroCross=off  InputSameDT=on
  Relational Operator2 : RelationalOperator  LogicOutDataTypeMode=boolean  OutDataTypeStr=boolean  ZeroCross=off  InputSameDT=on
  Sum : Sum  Inputs=++|  OutDataType=sfix(16)  OutScaling=2^0  RndMeth=Zero  SaturateOnIntegerOverflow=on  InputSameDT=on
  Sum1 : Sum  Inputs=++|  OutDataType=sfix(16)  OutScaling=2^0  RndMeth=Zero  SaturateOnIntegerOverflow=on  InputSameDT=on
  Switch : Switch  Criteria=u2 ~= 0  Threshold=1  RndMeth=Zero  ZeroCross=off  InputSameDT=on
  Switch1 : Switch  Criteria=u2 ~= 0  Threshold=1  RndMeth=Zero  ZeroCross=off  InputSameDT=on
  Terminator : Terminator
  Unit Delay : UnitDelay  SampleTime=-1
  Unit Delay1 : UnitDelay  SampleTime=-1
  Out : Outport
  wires:
  Logical Operator1/1 -> MotoHawk S-R Flip-Flop/2(R)
  Logical Operator2/1 -> MotoHawk S-R Flip-Flop/1(S)
  Relational Operator1/1 -> Logical Operator2/2
  Relational Operator2/1 -> Logical Operator1/2
  MotoHawk S-R Flip-Flop/2(!Q) -> Terminator/1
  MotoHawk S-R Flip-Flop/1(Q) -> Out/1
  Constant4/1 -> Relational Operator2/2
  Logical Operator/1 -> Logical Operator1/1, Switch1/2, Data Type Conversion1/1
  Data Type Conversion1/1 -> Sum1/2  "0 to 1"
  Sum1/1 -> Switch1/1  "0 to 65535 (saturate hi)"
  Constant3/1 -> Switch1/3
  Switch1/1 -> Relational Operator2/1, Unit Delay1/1  "0 to 65535"
  In/1 -> Logical Operator/1, Logical Operator2/1, Switch/2, Data Type Conversion/1
  Data Type Conversion/1 -> Sum/2  "0 to 1"
  Sum/1 -> Switch/1  "0 to 65535 (saturate hi)"
  Constant1/1 -> Switch/3
  Switch/1 -> Unit Delay/1, Relational Operator1/1  "0 to 65535"
  Constant2/1 -> Relational Operator1/2
  Unit Delay1/1 -> Sum1/1  "0 to 65535"
  Unit Delay/1 -> Sum/1  "0 to 65535"

== system BuckyWagon_01/Main Power Relay/Background/Post Shutdown two ticks before MPRD off ==
  Trigger : TriggerPort  TriggerType=falling
  Function-Call Generator : simulink/Ports & Subsystems/Function-Call Generator  sample_time=-1  numberOfIterations=1
  Post Shutdown two ticks before MPRD off : MotoHawk_lib/Trigger Blocks/motohawk_event_call  SystemSampleTime=-1  mode=Post Event  trigger=SHUTDOWN_EVENT  target=ECU565_128
  motohawk_code_coverage : MotoHawk_lib/Extra Development Blocks/motohawk_code_coverage
  wires:
  Function-Call Generator/1 -> Post Shutdown two ticks before MPRD off/Trigger

== system BuckyWagon_01/Main Power Relay/Background/Processor Reboot ==
  Enable : EnablePort
  Trigger : TriggerPort  TriggerType=falling
  Force Module Reset : MotoHawk_lib/Extra Development Blocks/Force Module Reset
  motohawk_code_coverage : MotoHawk_lib/Extra Development Blocks/motohawk_code_coverage

== system BuckyWagon_01/Main Power Relay/Background/Save NV Vars one tick before MPRD off ==
  Trigger : TriggerPort  TriggerType=falling
  Function-Call Generator : simulink/Ports & Subsystems/Function-Call Generator  sample_time=-1  numberOfIterations=1
  Save NV Vars one tick before MPRD off : MotoHawk_lib/Data Storage Blocks/motohawk_store_nvmem  SystemSampleTime=-1
  motohawk_code_coverage : MotoHawk_lib/Extra Development Blocks/motohawk_code_coverage
  wires:
  Function-Call Generator/1 -> Save NV Vars one tick before MPRD off/Trigger

== system BuckyWagon_01/Main Power Relay/Background/Shutdown power on ECU565-128 ==
  Trigger : TriggerPort  TriggerType=falling
  Function-Call Generator : simulink/Ports & Subsystems/Function-Call Generator  sample_time=-1  numberOfIterations=1
  Shutdown power on ECU565-128 : MotoHawk_lib/Extra Development Blocks/motohawk_shutdown_power  SystemSampleTime=-1
  motohawk_code_coverage : MotoHawk_lib/Extra Development Blocks/motohawk_code_coverage
  wires:
  Function-Call Generator/1 -> Shutdown power on ECU565-128/Trigger

== system BuckyWagon_01/Strategy/Actuators/A123 Battery Controller ==
  Contactor Command : Inport  OutDataType=sfix(16)  OutScaling=2^0
  Compare To Constant : simulink/Logic and Bit Operations/Compare To Constant  SystemSampleTime=-1  relop=>=  const=5  LogicOutDataTypeMode=uint8
  Emergency Power Off Comand : Constant  Value=0  OutDataTypeMode=uint8  OutDataType=fixdt(1, 16)  OutScaling=2^0  OutDataTypeStr=uint8
  Main Enable : Constant  OutDataTypeMode=uint8  OutDataType=fixdt(1, 16)  OutScaling=2^0  OutDataTypeStr=uint8
  Send CAN Messages3 : MotoHawk_lib/CAN Blocks/Send CAN Messages  bus=-2  nam='CAN_2'  msgl=BMS_A123_400  pace=5  labelwires=off
  Time Since Enabled (With Input)1 : motohawk_control_primitives_lib/Time Since Enabled (With Input)1  SystemSampleTime=-1  nam='A123_GroundFaultDetector_Enable_Timer'  samp_time=-1  init=0  upperlim=3600*24
  motohawk_override_abs5 : MotoHawk_lib/Calibration & Probing Blocks/motohawk_override_abs  SystemSampleTime=-1  parent_name='hsc_bcm_enable'  parent_val=0  show_more=on  name_source=Use Parameter  parent_read_level=1  parent_override_level=1  view_as=Number  enum_struct={'Disabled', 'Enabled'}  use_help_units=off  parent_help=''  parent_units=''  use_min_max=off  parent_min=-inf  parent_max=inf  use_precision=off  parent_precision=''  parent_gain=1  parent_offset=0  parent_exp=1  use_mototune_group=on  parent_group='Actuators | BCM'
  motohawk_override_abs6 : MotoHawk_lib/Calibration & Probing Blocks/motohawk_override_abs  SystemSampleTime=-1  parent_name='hsc_bcm_epo'  parent_val=0  show_more=on  name_source=Use Parameter  parent_read_level=1  parent_override_level=1  view_as=Number  enum_struct={'Disabled', 'Enabled'}  use_help_units=off  parent_help=''  parent_units=''  use_min_max=off  parent_min=-inf  parent_max=inf  use_precision=off  parent_precision=''  parent_gain=1  parent_offset=0  parent_exp=1  use_mototune_group=on  parent_group='Actuators | BCM'
  motohawk_override_abs7 : MotoHawk_lib/Calibration & Probing Blocks/motohawk_override_abs  SystemSampleTime=-1  parent_name='hsc_bcm_leakage_enable'  parent_val=0  show_more=on  name_source=Use Parameter  parent_read_level=1  parent_override_level=1  view_as=Number  enum_struct={'Disabled', 'Enabled'}  use_help_units=off  parent_help=''  parent_units=''  use_min_max=off  parent_min=-inf  parent_max=inf  use_precision=off  parent_precision=''  parent_gain=1  parent_offset=0  parent_exp=1  use_mototune_group=on  parent_group='Actuators | BCM'
  motohawk_override_abs8 : MotoHawk_lib/Calibration & Probing Blocks/motohawk_override_abs  SystemSampleTime=-1  parent_name='hsc_bcm_mainc_enable'  parent_val=0  show_more=on  name_source=Use Parameter  parent_read_level=1  parent_override_level=1  view_as=Number  enum_struct={'Disabled', 'Enabled'}  use_help_units=off  parent_help=''  parent_units=''  use_min_max=off  parent_min=-inf  parent_max=inf  use_precision=off  parent_precision=''  parent_gain=1  parent_offset=0  parent_exp=1  use_mototune_group=on  parent_group='Actuators | BCM'
  motohawk_probe6 : MotoHawk_lib/Calibration & Probing Blocks/motohawk_probe  nam='hsc_bcm_enable'  show_more=on  name_source=Use Parameter  read_level=1  view_as=Number  enum_struct={'Disabled', 'Enabled'}  vector_style=Wide Row  use_help_units=off  help=''  units=''  use_header_enum=off  row_header_enum={}  col_header_enum={}  use_precision=off  precision=''  gain=1  offset=0  exp=1  use_mototune_group=on  mototune_group='Actuators | BCM'
  motohawk_probe7 : MotoHawk_lib/Calibration & Probing Blocks/motohawk_probe  nam='hsc_bcm_epo'  show_more=on  name_source=Use Parameter  read_level=1  view_as=Number  enum_struct={'Disabled', 'Enabled'}  vector_style=Wide Row  use_help_units=off  help=''  units=''  use_header_enum=off  row_header_enum={}  col_header_enum={}  use_precision=off  precision=''  gain=1  offset=0  exp=1  use_mototune_group=on  mototune_group='Actuators | BCM'
  motohawk_probe8 : MotoHawk_lib/Calibration & Probing Blocks/motohawk_probe  nam='hsc_bcm_leakage_enable'  show_more=on  name_source=Use Parameter  read_level=1  view_as=Number  enum_struct={'Disabled', 'Enabled'}  vector_style=Wide Row  use_help_units=off  help=''  units=''  use_header_enum=off  row_header_enum={}  col_header_enum={}  use_precision=off  precision=''  gain=1  offset=0  exp=1  use_mototune_group=on  mototune_group='Actuators | BCM'
  motohawk_probe9 : MotoHawk_lib/Calibration & Probing Blocks/motohawk_probe  nam='hsc_bcm_mainc_enable'  show_more=on  name_source=Use Parameter  read_level=1  view_as=Number  enum_struct={'Disabled', 'Enabled'}  vector_style=Wide Row  use_help_units=off  help=''  units=''  use_header_enum=off  row_header_enum={}  col_header_enum={}  use_precision=off  precision=''  gain=1  offset=0  exp=1  use_mototune_group=on  mototune_group='Actuators | BCM'
  wires:
  motohawk_override_abs5/1 -> Send CAN Messages3/1
  motohawk_override_abs6/1 -> Send CAN Messages3/2
  motohawk_override_abs7/1 -> Send CAN Messages3/3
  motohawk_override_abs8/1 -> Send CAN Messages3/4
  Main Enable/1 -> motohawk_override_abs5/1, motohawk_probe6/1
  Emergency Power Off Comand/1 -> motohawk_override_abs6/1, motohawk_probe7/1
  Contactor Command/1 -> motohawk_override_abs8/1, motohawk_probe9/1, Time Since Enabled (With Input)1/1
  Compare To Constant/1 -> motohawk_override_abs7/1, motohawk_probe8/1
  Time Since Enabled (With Input)1/1 -> Compare To Constant/1

== system BuckyWagon_01/Strategy/Actuators/Brusa Charger ==
  In1 : Inport  OutDataType=sfix(16)  OutScaling=2^0
  Bus Selector : BusSelector  OutputSignals=CAN_Enable,ClearErrorLatch,ControlPilotVentReq,MaxMainsCurrent,OutputVoltageCommand,OutputCurrentCommand
  motohawk_override_abs{,1..2,4} (4 alike) : MotoHawk_lib/Calibration & Probing Blocks/motohawk_override_abs  SystemSampleTime=-1  parent_name='Override_Absolute'  parent_val=0  show_more=on  name_source=Use Output Wire Name  parent_read_level=1  parent_override_level=1  view_as=Number  enum_struct={'Disabled', 'Enabled'}  use_help_units=off  parent_help=''  parent_units=''  use_min_max=off  parent_min=-inf  parent_max=inf  use_precision=off  parent_precision=''  parent_gain=1  parent_offset=0  parent_exp=1  use_mototune_group=on  parent_group='Actuators | Brusa'
  motohawk_override_abs3 : MotoHawk_lib/Calibration & Probing Blocks/motohawk_override_abs  SystemSampleTime=-1  parent_name='Override_Absolute'  parent_val=0  show_more=on  name_source=Use Output Wire Name  parent_read_level=1  parent_override_level=1  view_as=Enumeration  enum_struct={'No Ventilation', 'Ventilation'}  use_help_units=off  parent_help=''  parent_units=''  use_min_max=off  parent_min=-inf  parent_max=inf  use_precision=off  parent_precision=''  parent_gain=1  parent_offset=0  parent_exp=1  use_mototune_group=on  parent_group='Actuators | Brusa'
  motohawk_override_abs5 : MotoHawk_lib/Calibration & Probing Blocks/motohawk_override_abs  SystemSampleTime=-1  parent_name='Override_Absolute'  parent_val=0  show_more=on  name_source=Use Output Wire Name  parent_read_level=1  parent_override_level=1  view_as=Enumeration  enum_struct={'Disabled', 'Enabled'}  use_help_units=off  parent_help=''  parent_units=''  use_min_max=off  parent_min=-inf  parent_max=inf  use_precision=off  parent_precision=''  parent_gain=1  parent_offset=0  parent_exp=1  use_mototune_group=on  parent_group='Actuators | Brusa'
  motohawk_probe{,1..2,4} (4 alike) : MotoHawk_lib/Calibration & Probing Blocks/motohawk_probe  nam='Probe'  show_more=on  name_source=Use Input Wire Name  read_level=1  view_as=Number  enum_struct={'Disabled', 'Enabled'}  vector_style=Wide Row  use_help_units=off  help=''  units=''  use_header_enum=off  row_header_enum={}  col_header_enum={}  use_precision=off  precision=''  gain=1  offset=0  exp=1  use_mototune_group=on  mototune_group='Actuators | Brusa'
  motohawk_probe3 : MotoHawk_lib/Calibration & Probing Blocks/motohawk_probe  nam='Probe'  show_more=on  name_source=Use Input Wire Name  read_level=1  view_as=Enumeration  enum_struct={'No Ventilation', 'Ventilation'}  vector_style=Wide Row  use_help_units=off  help=''  units=''  use_header_enum=off  row_header_enum={}  col_header_enum={}  use_precision=off  precision=''  gain=1  offset=0  exp=1  use_mototune_group=on  mototune_group='Actuators | Brusa'
  motohawk_probe5 : MotoHawk_lib/Calibration & Probing Blocks/motohawk_probe  nam='Probe'  show_more=on  name_source=Use Input Wire Name  read_level=1  view_as=Enumeration  enum_struct={'Disabled', 'Enabled'}  vector_style=Wide Row  use_help_units=off  help=''  units=''  use_header_enum=off  row_header_enum={}  col_header_enum={}  use_precision=off  precision=''  gain=1  offset=0  exp=1  use_mototune_group=on  mototune_group='Actuators | Brusa'
  wires:
  motohawk_override_abs5/1 -> motohawk_probe5/1  "CAN_Enable"
  motohawk_override_abs4/1 -> motohawk_probe4/1  "ClearErrorLtch"
  motohawk_override_abs3/1 -> motohawk_probe3/1  "CntrlPltVentReq"
  motohawk_override_abs2/1 -> motohawk_probe2/1  "MaxMainsCrnt"
  motohawk_override_abs1/1 -> motohawk_probe1/1  "OutVoltCmd"
  motohawk_override_abs/1 -> motohawk_probe/1  "OutCrntCmd"
  Bus Selector/1 -> motohawk_override_abs5/1  "<CAN_Enable>"
  Bus Selector/2 -> motohawk_override_abs4/1  "<ClearErrorLatch>"
  Bus Selector/3 -> motohawk_override_abs3/1  "<ControlPilotVentReq>"
  Bus Selector/4 -> motohawk_override_abs2/1  "<MaxMainsCurrent>"
  Bus Selector/5 -> motohawk_override_abs1/1  "<OutputVoltageCommand>"
  Bus Selector/6 -> motohawk_override_abs/1  "<OutputCurrentCommand>"
  In1/1 -> Bus Selector/1

== system BuckyWagon_01/Strategy/Actuators/Cruise Control Indicator ==
  Chart : Stateflow chart  TreatAsAtomicUnit=on
  motohawk_calibration1 : MotoHawk_lib/Calibration & Probing Blocks/motohawk_calibration  nam='cCInd_ShortTime'  val=20  storage=Calibration  show_more=on  name_source=Use Parameter  data_type=uint16  read_level=1  write_level=1  ovr_cals=on  view_as=Number  enum_struct={'Disabled', 'Enabled'}  vector_style=Wide Row  use_help_units=on  help='Short Off time in sequence.'  units='s'  use_header_enum=off  row_header_enum={}  col_header_enum={}  use_min_max=on  min_val=0  max_val=100  use_precision=on  precision='1.3'  gain=0.005  offset=0  exp=1  use_mototune_group=off  mototune_group=motohawk_vardec_path(gcb)
  motohawk_calibration2 : MotoHawk_lib/Calibration & Probing Blocks/motohawk_calibration  nam='cCInd_LongOff'  val=300  storage=Calibration  show_more=on  name_source=Use Parameter  data_type=uint16  read_level=1  write_level=1  ovr_cals=on  view_as=Number  enum_struct={'Disabled', 'Enabled'}  vector_style=Wide Row  use_help_units=on  help='Long Off time in flash sequence.'  units='s'  use_header_enum=off  row_header_enum={}  col_header_enum={}  use_min_max=on  min_val=0  max_val=100  use_precision=on  precision='1.3'  gain=0.005  offset=0  exp=1  use_mototune_group=off  mototune_group=motohawk_vardec_path(gcb)
  motohawk_calibration3 : MotoHawk_lib/Calibration & Probing Blocks/motohawk_calibration  nam='cCInd_OnTime'  val=10  storage=Calibration  show_more=on  name_source=Use Parameter  data_type=uint16  read_level=1  write_level=1  ovr_cals=on  view_as=Number  enum_struct={'Disabled', 'Enabled'}  vector_style=Wide Row  use_help_units=on  help='On time in flash sequence.'  units='s'  use_header_enum=off  row_header_enum={}  col_header_enum={}  use_min_max=on  min_val=0  max_val=100  use_precision=on  precision='1.3'  gain=0.005  offset=0  exp=1  use_mototune_group=off  mototune_group=motohawk_vardec_path(gcb)
  motohawk_data_read : MotoHawk_lib/Data Storage Blocks/motohawk_data_read  source=Lookup By Name  structure=Scalar  operation=Read scalar from location by index  sz_vec=4  sz_row=2  sz_col=3  typ=uint8  nam='cCOn'  checkNull=on  struct_inst_name=''  struct_nam='MyStruct'
  Out : Outport  OutDataType=sfix(16)  OutScaling=2^0
  wires:
  motohawk_data_read/1 -> Chart/1(cCOn)
  motohawk_calibration2/1 -> Chart/2(offLongTime)
  motohawk_calibration1/1 -> Chart/3(offShortTime)
  motohawk_calibration3/1 -> Chart/4(onTime)
  Chart/1(light) -> Out/1

== system BuckyWagon_01/Strategy/Actuators/DC/DC Converter Controller ==
  Enable : Inport  DataType=boolean  OutDataType=sfix(16)  OutScaling=2^0  OutDataTypeStr=boolean
  Discrete Actuator Characterization1 : motohawk_engine_lib/Discrete Actuator Characterization  SystemSampleTime=-1  prefix='InhibitDCDC_Out_'  nam='InhibitDCDC_Out'  units='bool'  parent_group='Actuators | DC/DC'  polarity=Low-True
  Logical Operator : Logic  Operator=NOT  Inputs=1  AllPortsSameDT=off  OutDataTypeMode=boolean  LogicDataType=fixdt(0, 8)  OutDataTypeStr=boolean
  motohawk_dout1 : MotoHawk_lib/Digital I//O Blocks/motohawk_dout  resource_name=[]  text_resource=LSD6  target=ECU565-128  use_diag=off  use_vardec=on  nam='DCDCInhibit_Out_Pin'  read_level=1  write_level=1  group='System | I/O Pins | Outputs Config'
  wires:
  Discrete Actuator Characterization1/1 -> motohawk_dout1/1
  Enable/1 -> Logical Operator/1
  Logical Operator/1 -> Discrete Actuator Characterization1/1
